simulink model "G_Sim_V2"  (R2024b)
settings: Solver=VariableStepAuto  StartTime=0.0  StopTime=0.006  MaxStep=10e-9  RelTol=1e-3
libraries: dspxfrm3 x1, dspmlti4 x1, dspsigops x1
settings Model: SimulationMode=accelerator  PacingRate=1000  Creator=Lenovo  LastModifiedBy=Lenovo

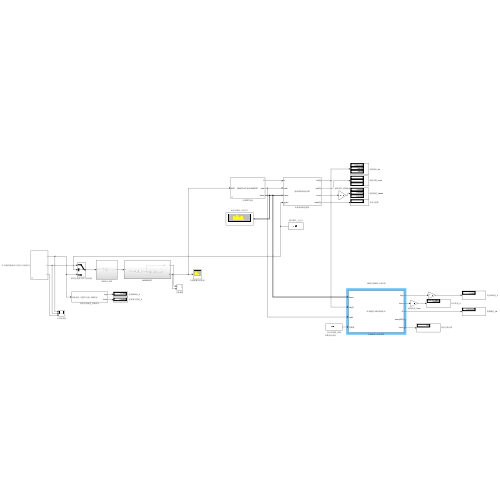
[thumbnail: Simulink's stored preview of the top-level diagram]
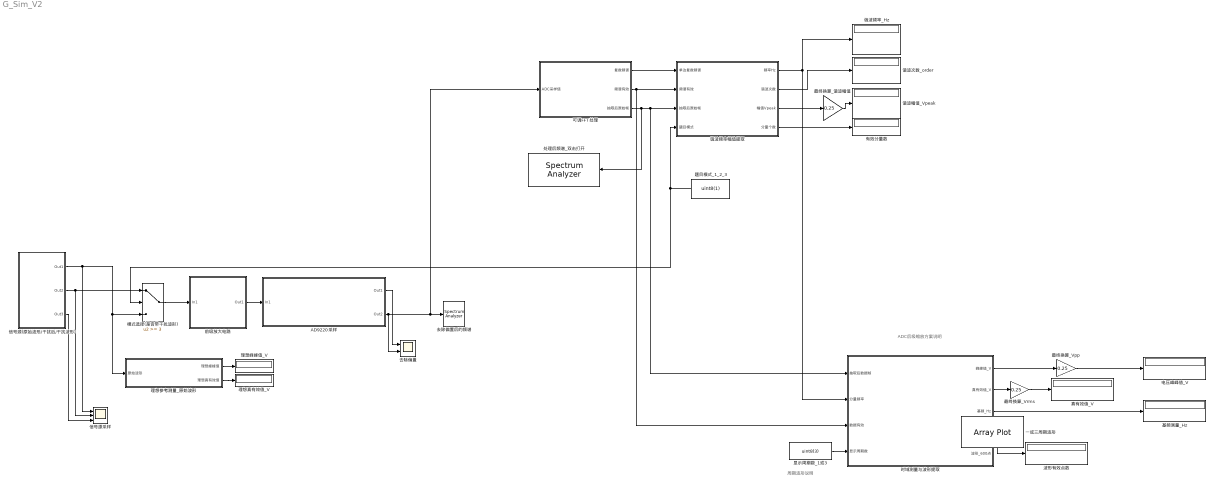
== system G_Sim_V2 ==
  note: 周期波形说明
  note: ADC后级缩放方案说明
  AD9220采样 : Subsystem
  信号源(原始波形/干扰后/干扰波形) : Subsystem  mask{frequency=50e3, harmonic_order_a=3, harmonic_order_b=4, amplitude_0=60e-3, harmonic_amplitude_a=30e-3, harmonic_amplitude_b=15e-3}
      mask DialogControl Param Prompt: Param
  信号源采样 : Scope  NumInputPorts=3
  前级放大电路 : Subsystem
  去除偏置 : Scope  NumInputPorts=2
  去除偏置后的频谱 : SpectrumAnalyzer  WindowPosition=[18.000000,282.000000,800.000000,500.000000,]  ScopeFrameLocation=window  Method=Welch  PlotAsTwoSidedSpectrum=off  FrequencyScale=Log  AveragingMethod=Exponential  YLimits=[-230.71408163,41.60076026]  ColorLimits=[-227.89340735,34.77530027]  SelectedToolstripTab=spectrumAnalyzerToolstrip.measurementsTab
  可调FFT处理 : Subsystem  mask{Fs=2e6, NFFT=4096, FsADC=8e6, Decimation=4}
      mask prompts: Fs "处理采样率 Fs (Hz)"; NFFT "FFT点数 NFFT"; FsADC "ADC采样率 FsADC (Hz)"; Decimation "抽取倍数"
      mask Display:
      | disp('8M采样/4倍抽取/4096FFT');
      | port_label('input',1,'ADC');
      | port_label('output',1,'X');
      | port_label('output',2,'valid');
      | port_label('output',3,'frame');
  基频测量_Hz : Display
  处理后频谱_双击打开 : SpectrumAnalyzer  WindowPosition=[13.000000,137.000000,800.000000,500.000000,]  ScopeFrameLocation=window  Method=Welch  PlotAsTwoSidedSpectrum=off  FrequencyScale=Log  AveragingMethod=Exponential  YLimits=[-134.74840915,29.25983367]  ColorLimits=[-227.89340735,34.77530027]  SelectedToolstripTab=spectrumAnalyzerToolstrip.measurementsTab
  时域测量与波形提取 : Subsystem
      mask Display:
      | disp('时域测量/1或3周期波形');
      | port_label('input',1,'frame');
      | port_label('input',2,'Hz[3]');
      | port_label('input',3,'valid');
      | port_label('input',4,'周期数');
      | port_label('output',1,'Vpp');
      | port_label('output',2,'Vrms');
      | port_label('output',3,'f0');
      | port_label('output',4,'wave[600]');
      | port_label('output',5,'count');
  显示周期数_1或3 : Constant  Value=uint8(3)  OutDataTypeStr=uint8
  最终换算_Vpp : Gain  Gain=0.25
  最终换算_Vrms : Gain  Gain=0.25
  最终换算_谐波幅值 : Gain  Gain=0.25
  有效分量数 : Display
  模式选择(是否带干扰波形) : Switch  Threshold=3  SaturateOnIntegerOverflow=off  InputSameDT=off
  波形有效点数 : Display
  理想参考测量_原始波形 : Subsystem
      mask Display:
      | disp('理想参考值（ADC前）');
      | port_label('input',1,'原始波形');
      | port_label('output',1,'Vpp');
      | port_label('output',2,'Vrms');
  理想峰峰值_V : Display
  理想真有效值_V : Display
  电压峰峰值_V : Display
  真有效值_V : Display
  谐波幅值_Vpeak : Display
  谐波次数_order : Display
  谐波频率_Hz : Display
  谐波频率幅值提取 : Subsystem  mask{Fs=2e6, NFFT=4096, MinFreq=10e3, MaxFreq=500e3, MinAmp=4e-3}
      mask prompts: Fs "采样率 Fs (Hz)"; NFFT "FFT点数 NFFT"; MinFreq "最低分析频率 (Hz)"; MaxFreq "最高分析频率 (Hz)"; MinAmp "最小有效幅值 (Vpeak)"
      mask Display:
      | disp('谐波频率/幅值/次数');
      | port_label('input',1,'X');
      | port_label('input',2,'valid');
      | port_label('input',3,'frame');
      | port_label('input',4,'mode');
      | port_label('output',1,'Hz[3]');
      | port_label('output',2,'Vpk[3]');
      | port_label('output',3,'count');
      | port_label('output',4,'order[3]');
  题目模式_1_2_3 : Constant  Value=uint8(1)  OutDataTypeStr=uint8
  一或三周期波形 : ArrayPlot  IOType=viewer  IsFloating=on  WindowPosition=[82.000000,136.000000,800.000000,500.000000,]  ScopeFrameLocation=window  YLimits=[-0.6245688618118564 0.5422762307264692]  DefaultConfigurationName=dsp.scopes.ArrayPlotBlockSpecification
  wires:
  谐波频率幅值提取/1(频率Hz) -> 时域测量与波形提取/2(分量频率), 谐波频率_Hz/1
  谐波频率幅值提取/4(分量个数) -> 有效分量数/1
  可调FFT处理/1(复数频谱) -> 谐波频率幅值提取/1(单边复数频谱)
  可调FFT处理/2(频谱有效) -> 谐波频率幅值提取/2(频谱有效), 时域测量与波形提取/3(数据有效)
  可调FFT处理/3(抽取后原始帧) -> 时域测量与波形提取/1(抽取后数据帧), 谐波频率幅值提取/3(抽取后原始帧), 处理后频谱_双击打开/1
  题目模式_1_2_3/1 -> 模式选择(是否带干扰波形)/2, 谐波频率幅值提取/4(题目模式)
  显示周期数_1或3/1 -> 时域测量与波形提取/4(显示周期数)
  时域测量与波形提取/3(基频_Hz) -> 基频测量_Hz/1
  时域测量与波形提取/4(波形有效点数) -> 波形有效点数/1
  信号源(原始波形/干扰后/干扰波形)/1(Out1) -> 理想参考测量_原始波形/1(原始波形), 模式选择(是否带干扰波形)/3, 信号源采样/1
  信号源(原始波形/干扰后/干扰波形)/2(Out2) -> 模式选择(是否带干扰波形)/1, 信号源采样/2
  信号源(原始波形/干扰后/干扰波形)/3(Out3) -> 信号源采样/3
  谐波频率幅值提取/2(谐波次数) -> 谐波次数_order/1
  理想参考测量_原始波形/1(理想峰峰值) -> 理想峰峰值_V/1
  理想参考测量_原始波形/2(理想真有效值) -> 理想真有效值_V/1
  谐波频率幅值提取/3(幅值Vpeak) -> 最终换算_谐波幅值/1
  最终换算_谐波幅值/1 -> 谐波幅值_Vpeak/1
  时域测量与波形提取/1(峰峰值_V) -> 最终换算_Vpp/1
  最终换算_Vpp/1 -> 电压峰峰值_V/1
  时域测量与波形提取/2(真有效值_V) -> 最终换算_Vrms/1
  最终换算_Vrms/1 -> 真有效值_V/1
  模式选择(是否带干扰波形)/1 -> 前级放大电路/1(In1)
  AD9220采样/2(Out2) -> 可调FFT处理/1(ADC采样值), 去除偏置后的频谱/1, 去除偏置/2
  前级放大电路/1(Out1) -> AD9220采样/1(In1)
  AD9220采样/1(Out1) -> 去除偏置/1

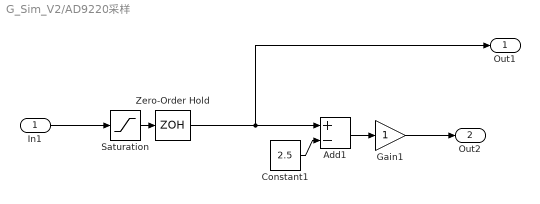
== system G_Sim_V2/AD9220采样 ==
  In1 : Inport
  Add1 : Sum  Inputs=+-
  Constant1 : Constant  Value=2.5
  Gain1 : Gain
  Saturation : Saturate  UpperLimit=5  LowerLimit=0
  Zero-Order Hold : ZeroOrderHold  SampleTime=1/8e6
  Out1 : Outport
  Out2 : Outport  Port=2
  wires:
  Add1/1 -> Gain1/1
  Saturation/1 -> Zero-Order Hold/1
  Constant1/1 -> Add1/2
  Gain1/1 -> Out2/1
  Zero-Order Hold/1 -> Out1/1, Add1/1
  In1/1 -> Saturation/1

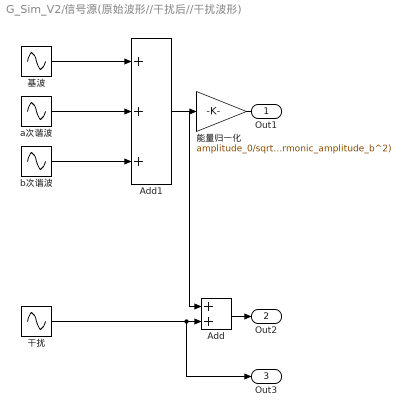
== system G_Sim_V2/信号源(原始波形//干扰后//干扰波形) ==
  Add : Sum
  Add1 : Sum  Inputs=+++
  能量归一化 : Gain  Gain=amplitude_0/sqrt(amplitude_0^2+harmonic_amplitude_a^2+harmonic_amplitude_b^2)
  a次谐波 : Sin  Amplitude=harmonic_amplitude_a  Frequency=2*pi*frequency*harmonic_order_a  SampleTime=0
  b次谐波 : Sin  Amplitude=harmonic_amplitude_b  Frequency=2*pi*frequency*harmonic_order_b  SampleTime=0
  基波 : Sin  Amplitude=amplitude_0  Frequency=2*pi*frequency  SampleTime=0
  干扰 : Sin  Amplitude=100e-3  Frequency=2*pi*1.2e6  SampleTime=0
  Out1 : Outport
  Out2 : Outport  Port=2
  Out3 : Outport  Port=3
  wires:
  a次谐波/1 -> Add1/2
  b次谐波/1 -> Add1/3
  基波/1 -> Add1/1
  Add1/1 -> 能量归一化/1
  能量归一化/1 -> Add/1, Out1/1
  干扰/1 -> Out3/1, Add/2
  Add/1 -> Out2/1

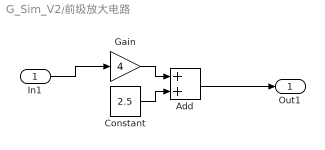
== system G_Sim_V2/前级放大电路 ==
  In1 : Inport
  Add : Sum
  Constant : Constant  Value=2.5
  Gain : Gain  Gain=4
  Out1 : Outport
  wires:
  In1/1 -> Gain/1
  Constant/1 -> Add/2
  Add/1 -> Out1/1
  Gain/1 -> Add/1

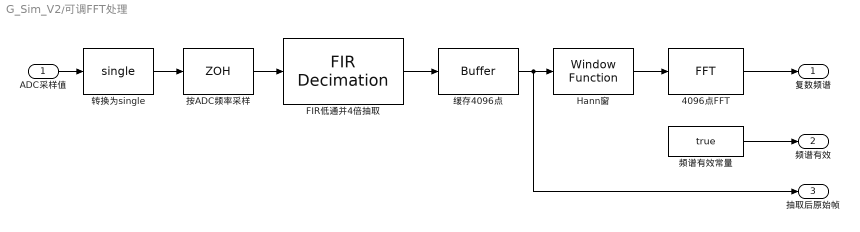
== system G_Sim_V2/可调FFT处理 ==
  ADC采样值 : Inport
  4096点FFT : dspxfrm3/FFT  FFTImplementation=Auto  CompMethod=Table lookup  TableOpt=NEW  TableOptActive=Speed  BitRevOrder=off  Normalize=off  InheritFFTLength=on  FFTLength=64  WrapInput=on  roundingMode=Ceiling  overflowMode=off  firstCoeffDataTypeStr=Inherit: Same word length as input  firstCoeffLastDataTypeStr=Inherit: Same word length as input  outputMin=[]  outputMax=[]
  FIR低通并4倍抽取 : dspmlti4/FIR Decimation  FilterSource=Dialog parameters  h=[-1.093832325746845e-05 -6.292254736687438e-05 -0.0001456190566409851 -0.000210121213955772 -0.0001715204318703031 5.201786070564381e-05 0.0004740892277420891 0.0009791364033496543 0.001309961916795507 0.001139443592884425 0.0002271750021134837 -0.001389645221210771 -0.00326542298539904 -0.004577381356277919 -0.004374292500219585 -0.00200400120335077 0.00242713788631572 0.00778010462815952 0.01199664830895183 0.01268492551912718 0.00806980856872996 -0.001995124150862495 -0.01536663043623436 -0.02767001830927002 -0.03323335274731441 -0.02673559895993285 -0.005096036961720372 0.03104031203495614 0.07681183656132551 0.1239468431957101 0.1627378137916923 0.184631371906325 0.184631371906325 0.1627378137916923 0.1239468431957101 0.07681183656132551 0.03104031203495614 -0.005096036961720372 -0.02673559895993285 -0.03323335274731441 -0.02767001830927002 -0.01536663043623436 -0.001995124150862495 0.00806980856872996 0.01268492551912718 0.01199664830895183 0.00778010462815952 0.00242713788631572 -0.00200400120335077 -0.004374292500219585 -0.004577381356277919 -0.00326542298539904 -0.001389645221210771 0.0002271750021134837 0.001139443592884425 0.001309961916795507 0.0009791364033496543 0.0004740892277420891 5.201786070564381e-05 -0.0001715204318703031 -0.000210121213955772 -0.0001456190566409851 -6.292254736687438e-05 -1.093832325746845e-05]  D=Decimation  filtStruct=Direct form transposed  FilterObject=FDECIM  framing=Allow multirate processing  AllowArbitraryInputLength=off  inputOffset=0  outputBufInitCond=0  roundingMode=Floor  overflowMode=off  firstCoeffDataTypeStr=Inherit: Same word length as input  firstCoeffMin=[]  firstCoeffMax=[]  firstCoeffLastDataTypeStr=Inherit: Same word length as input  outputDataTypeStr=Inherit: Same as accumulator  outputMin=[]  outputMax=[]  outputLastDataTypeStr=Inherit: Same as accumulator
  Hann窗 : dspsigops/Window Function  winmode=Apply window to input  wintype=Hann  sampmode=Discrete  samptime=1  N=64  Rs=50  beta=10  winsamp=Symmetric  UserWindow=hamming  OptParams=off  UserParams={'symmetric'}  dataType=double  isSigned=on  wordLen=16  udDataType=sfix(16)  fracBitsMode=Best precision  numFracBits=15  roundingMode=Floor  overflowMode=off  numSidelobes=4  sidelobeLevel=-30
  按ADC频率采样 : ZeroOrderHold  SampleTime=1/FsADC
  缓存4096点 : Buffer  N=NFFT
  转换为single : DataTypeConversion  OutDataTypeStr=single  SaturateOnIntegerOverflow=off  RndMeth=Floor
  频谱有效常量 : Constant  Value=true  OutDataTypeStr=boolean  SampleTime=NFFT/Fs
  复数频谱 : Outport
  频谱有效 : Outport  Port=2
  抽取后原始帧 : Outport  Port=3
  wires:
  ADC采样值/1 -> 转换为single/1
  转换为single/1 -> 按ADC频率采样/1
  按ADC频率采样/1 -> FIR低通并4倍抽取/1
  FIR低通并4倍抽取/1 -> 缓存4096点/1
  缓存4096点/1 -> Hann窗/1, 抽取后原始帧/1
  Hann窗/1 -> 4096点FFT/1
  4096点FFT/1 -> 复数频谱/1
  频谱有效常量/1 -> 频谱有效/1

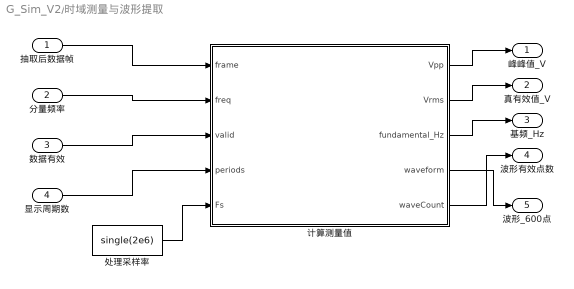
== system G_Sim_V2/时域测量与波形提取 ==
  抽取后数据帧 : Inport
  分量频率 : Inport  Port=2
  数据有效 : Inport  Port=3
  显示周期数 : Inport  Port=4
  处理采样率 : Constant  Value=single(2e6)  OutDataTypeStr=single
  计算测量值 : MATLAB Function  TreatAsAtomicUnit=on
  峰峰值_V : Outport
  真有效值_V : Outport  Port=2
  基频_Hz : Outport  Port=3
  波形有效点数 : Outport  Port=4
  波形_600点 : Outport  Port=5
  wires:
  抽取后数据帧/1 -> 计算测量值/1(frame)
  分量频率/1 -> 计算测量值/2(freq)
  数据有效/1 -> 计算测量值/3(valid)
  显示周期数/1 -> 计算测量值/4(periods)
  处理采样率/1 -> 计算测量值/5(Fs)
  计算测量值/1(Vpp) -> 峰峰值_V/1
  计算测量值/2(Vrms) -> 真有效值_V/1
  计算测量值/3(fundamental_Hz) -> 基频_Hz/1
  计算测量值/4(waveform) -> 波形_600点/1
  计算测量值/5(waveCount) -> 波形有效点数/1

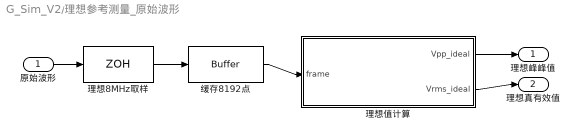
== system G_Sim_V2/理想参考测量_原始波形 ==
  原始波形 : Inport
  理想8MHz取样 : ZeroOrderHold  SampleTime=1/8e6
  理想值计算 : MATLAB Function  TreatAsAtomicUnit=on
  缓存8192点 : Buffer  N=8192
  理想峰峰值 : Outport
  理想真有效值 : Outport  Port=2
  wires:
  原始波形/1 -> 理想8MHz取样/1
  理想8MHz取样/1 -> 缓存8192点/1
  缓存8192点/1 -> 理想值计算/1(frame)
  理想值计算/1(Vpp_ideal) -> 理想峰峰值/1
  理想值计算/2(Vrms_ideal) -> 理想真有效值/1

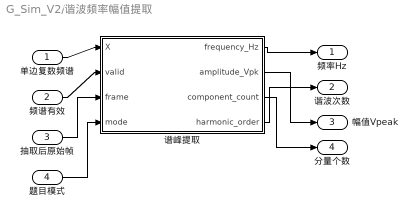
== system G_Sim_V2/谐波频率幅值提取 ==
  单边复数频谱 : Inport
  频谱有效 : Inport  Port=2
  抽取后原始帧 : Inport  Port=3
  题目模式 : Inport  Port=4
  谱峰提取 : MATLAB Function  TreatAsAtomicUnit=on
  频率Hz : Outport
  谐波次数 : Outport  Port=2
  幅值Vpeak : Outport  Port=3
  分量个数 : Outport  Port=4
  wires:
  单边复数频谱/1 -> 谱峰提取/1(X)
  频谱有效/1 -> 谱峰提取/2(valid)
  谱峰提取/1(frequency_Hz) -> 频率Hz/1
  谱峰提取/2(amplitude_Vpk) -> 幅值Vpeak/1
  谱峰提取/3(component_count) -> 分量个数/1
  抽取后原始帧/1 -> 谱峰提取/3(frame)
  题目模式/1 -> 谱峰提取/4(mode)
  谱峰提取/4(harmonic_order) -> 谐波次数/1

== matlab function G_Sim_V2/谐波频率幅值提取/谱峰提取 ==
  data: X input; frequency_Hz output; valid input; frame input; mode input; amplitude_Vpk output; component_count output; Fs parameter; NFFT parameter; MinFreq parameter; MaxFreq parameter; MinAmp parameter; harmonic_order output
function [frequency_Hz, amplitude_Vpk, component_count, harmonic_order] = fcn(X, valid, frame, mode, Fs, NFFT, MinFreq, MaxFreq, MinAmp)
%#codegen
N=coder.const(NFFT);
frequency_Hz=zeros(3,1,'single');
amplitude_Vpk=zeros(3,1,'single');
component_count=uint8(0);
harmonic_order=zeros(3,1,'uint8');
if ~valid
    return;
end
mag=abs(X);
k0=max(2,ceil(MinFreq*N/Fs)+1);
if mode==1
    maxF=single(200e3);
else
    maxF=single(500e3);
end
k1=min(N/2,ceil(double(maxF)*N/Fs)+2);
bestScore=zeros(3,1,'single');
bestBin=zeros(3,1,'single');
for k=k0:k1
    if mag(k)>=mag(k-1) && mag(k)>mag(k+1)
        y1=log(max(mag(k-1),single(1e-30)));
        y2=log(max(mag(k),single(1e-30)));
        y3=log(max(mag(k+1),single(1e-30)));
        den=y1-2*y2+y3;
        delta=single(0);
        if abs(den)>single(1e-20)
            delta=single(0.5)*(y1-y3)/den;
        end
        delta=min(single(0.5),max(single(-0.5),delta));
        ampApprox=single(2)*(mag(k-1)+mag(k)+mag(k+1))/single(N-1);
        if ampApprox>=single(MinAmp)
            for j=1:3
                if ampApprox>bestScore(j)
                    for q=3:-1:j+1
                        bestScore(q)=bestScore(q-1); bestBin(q)=bestBin(q-1);
                    end
                    bestScore(j)=ampApprox; bestBin(j)=single(k-1)+delta;
                    break;
                end
            end
        end
    end
end
for j=1:3
    if bestScore(j)>0
        frequency_Hz(j)=bestBin(j)*single(Fs/N);
        component_count=component_count+1;
    end
end
for a=1:2
    for bidx=a+1:3
        if frequency_Hz(bidx)>0 && (frequency_Hz(a)==0 || frequency_Hz(bidx)<frequency_Hz(a))
            tf=frequency_Hz(a); frequency_Hz(a)=frequency_Hz(bidx); frequency_Hz(bidx)=tf;
        end
    end
end
% Calculate harmonic order from frequency ratio to the fundamental.
if frequency_Hz(1)>0
    for j=1:3
        if frequency_Hz(j)>0
            ratio=frequency_Hz(j)/frequency_Hz(1);
            orderValue=round(ratio);
            if orderValue>=1 && orderValue<=255 && abs(ratio-orderValue)<single(0.15)
                harmonic_order(j)=uint8(orderValue);
            end
        end
    end
end
dc=single(0);
for n=1:N
    dc=dc+frame(n);
end
dc=dc/single(N);
for j=1:3
    f=frequency_Hz(j);
    if f>0
        omega=single(2*pi)*f/single(Fs);
        cw=cos(omega); sw=sin(omega);
        c=single(1); s=single(0);
        cc=single(0); ss=single(0); cs=single(0); yc=single(0); ys=single(0);
        for n=1:N
            y=frame(n)-dc;
            cc=cc+c*c; ss=ss+s*s; cs=cs+c*s;
            yc=yc+y*c; ys=ys+y*s;
            cn=c*cw-s*sw; sn=s*cw+c*sw; c=cn; s=sn;
            if bitand(n,255)==0
                r=sqrt(c*c+s*s); c=c/r; s=s/r;
            end
        end
        detv=cc*ss-cs*cs;
        if abs(detv)>single(1e-20)
            ac=(yc*ss-ys*cs)/detv;
            as=(ys*cc-yc*cs)/detv;
            amplitude_Vpk(j)=sqrt(ac*ac+as*as);
        end
    end
end
end

== matlab function G_Sim_V2/时域测量与波形提取/计算测量值 ==
  data: frame input; Vpp output; freq input; valid input; periods input; Fs input; Vrms output; fundamental_Hz output; waveform output; waveCount output
function [Vpp, Vrms, fundamental_Hz, waveform, waveCount] = fcn(frame, freq, valid, periods, Fs)
%#codegen
MAX_POINTS = 600;
waveform = zeros(MAX_POINTS,1,'single');
Vpp = single(0);
Vrms = single(0);
fundamental_Hz = single(0);
waveCount = uint16(0);
if ~valid
    return;
end
N = numel(frame);
dc = single(0);
for n = 1:N
    dc = dc + frame(n);
end
dc = dc / single(N);
energy = single(0);
imax = 1;
imin = 1;
ymax = frame(1) - dc;
ymin = ymax;
for n = 1:N
    y = frame(n) - dc;
    energy = energy + y*y;
    if y > ymax
        ymax = y; imax = n;
    end
    if y < ymin
        ymin = y; imin = n;
    end
end
Vrms = sqrt(energy / single(N));
% Three-point parabolic interpolation corrects peaks between ADC samples.
ymax = peak_vertex(frame, dc, imax, N, true);
ymin = peak_vertex(frame, dc, imin, N, false);
Vpp = ymax - ymin;
fundamental_Hz = freq(1);
if fundamental_Hz <= 0
    return;
end
samplesPerPeriod = max(1, round(double(Fs) / double(fundamental_Hz)));
p = min(3, max(1, double(periods)));
count = min(MAX_POINTS, p*samplesPerPeriod);
startIndex = 1;
for n = 2:(N-count)
    if frame(n-1)-dc <= 0 && frame(n)-dc > 0
        startIndex = n;
        break;
    end
end
for n = 1:count
    waveform(n) = frame(startIndex+n-1) - dc;
end
waveCount = uint16(count);
end

function yv = peak_vertex(x, dc, k, N, isMaximum)
%#codegen
km = k-1; if km < 1, km = N; end
kp = k+1; if kp > N, kp = 1; end
ym = x(km)-dc; y0 = x(k)-dc; yp = x(kp)-dc;
den = single(8)*(yp+ym-single(2)*y0);
yv = y0;
if abs(den) > single(1e-12)
    candidate = y0 - (yp-ym)*(yp-ym)/den;
    if (isMaximum && candidate >= y0) || (~isMaximum && candidate <= y0)
        yv = candidate;
    end
end
end

== matlab function G_Sim_V2/理想参考测量_原始波形/理想值计算 ==
  data: frame input; Vpp_ideal output; Vrms_ideal output
function [Vpp_ideal, Vrms_ideal] = fcn(frame)
%#codegen
N=numel(frame);
dc=single(0);
for n=1:N
    dc=dc+single(frame(n));
end
dc=dc/single(N);
energy=single(0);
imax=1; imin=1;
ymax=single(frame(1))-dc;
ymin=ymax;
for n=1:N
    y=single(frame(n))-dc;
    energy=energy+y*y;
    if y>ymax, ymax=y; imax=n; end
    if y<ymin, ymin=y; imin=n; end
end
Vrms_ideal=sqrt(energy/single(N));
ymax=vertex(frame,dc,imax,N,true);
ymin=vertex(frame,dc,imin,N,false);
Vpp_ideal=ymax-ymin;
end

function yv=vertex(x,dc,k,N,isMax)
%#codegen
km=k-1; if km<1, km=N; end
kp=k+1; if kp>N, kp=1; end
ym=single(x(km))-dc; y0=single(x(k))-dc; yp=single(x(kp))-dc;
den=single(8)*(yp+ym-single(2)*y0);
yv=y0;
if abs(den)>single(1e-12)
    candidate=y0-(yp-ym)*(yp-ym)/den;
    if (isMax && candidate>=y0) || (~isMax && candidate<=y0)
        yv=candidate;
    end
end
end
